simulink model "NonLineare"  (R2020b)
settings: Solver=ode45  StartTime=0.0  StopTime=100  RelTol=1e-6
values from neighbouring files (symbols this model uses):
  alpha = 1    [Assignment7Mat.m]
  C_te = [1 0 0 0]    [Assignment7Mat.m]
  d1_amp = 0.5    [Assignment7Mat.m]
  d1_period = 50    [Assignment7Mat.m]
  F = 1    [Assignment7Mat.m]
  g = 9.81    [Assignment7Mat.m]
  K = -ack*pDesA    [Assignment7Mat.m]
  l = 1    [Assignment7Mat.m]
  L = Gamma - K*Pi    [Assignment7Mat.m]
  M = 1    [Assignment7Mat.m]
  omega = 0.1    [Assignment7Mat.m]
  Q_te = [-1 0 0]    [Assignment7Mat.m]
  x0 = [0 0 0 0]    [Assignment7Mat.m]
settings Model: Creator=Paolo  LastModifiedBy=Paolo

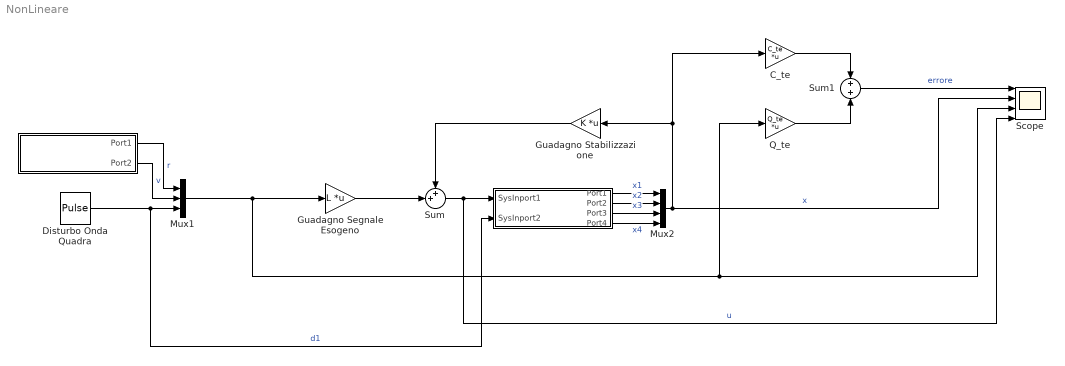
== system NonLineare ==
  "  " : Subsystem  mask(Differential Equation Editor (DEE)){}
      settings: OpenFcn=diffeqed
      mask Display: disp('ModelloNonLineare')
  "   " : Subsystem  mask(Differential Equation Editor (DEE)){}
      settings: OpenFcn=diffeqed
      mask Display: disp('Sistema Esogeno')
  C_te : Gain  Gain=C_te  Multiplication=Matrix(K*u)
  Disturbo Onda Quadra : DiscretePulseGenerator  PulseType=Time based  Amplitude=d1_amp  Period=d1_period  PulseWidth=50
  Guadagno Stabilizzazione : Gain  Gain=K  Multiplication=Matrix(K*u)
  Guadagno Segnale Esogeno : Gain  Gain=L  Multiplication=Matrix(K*u)
  Mux1 : Mux  Inputs=3
  Mux2 : Mux
  Q_te : Gain  Gain=Q_te  Multiplication=Matrix(K*u)
  Scope : Scope  NumInputPorts=4
  Sum : Sum  Inputs=++|
  Sum1 : Sum  Inputs=+|+
  wires:
  Mux2/1 -> C_te/1, Guadagno Stabilizzazione/1, Scope/2  "x"
  "   "/2(Port2) -> Mux1/2  "v"
  Guadagno Stabilizzazione/1 -> Sum/1
  Mux1/1 -> Scope/3, Q_te/1, Guadagno Segnale Esogeno/1
  Guadagno Segnale Esogeno/1 -> Sum/2
  C_te/1 -> Sum1/1
  Sum1/1 -> Scope/1  "errore"
  Sum/1 -> "  "/1(SysInport1), Scope/4  "u"
  Q_te/1 -> Sum1/2
  "   "/1(Port1) -> Mux1/1  "r"
  Disturbo Onda Quadra/1 -> "  "/2(SysInport2), Mux1/3  "d1"
  "  "/1(Port1) -> Mux2/1  "x1"
  "  "/2(Port2) -> Mux2/2  "x2"
  "  "/4(Port4) -> Mux2/4  "x4"
  "  "/3(Port3) -> Mux2/3  "x3"

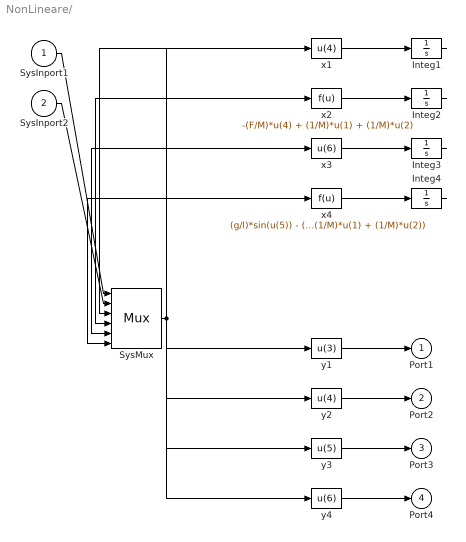
== system NonLineare/   ==
  SysInport1 : Inport
  SysInport2 : Inport  Port=2
  Integ1 : Integrator  InitialCondition=x0(1)
  Integ2 : Integrator  InitialCondition=x0(2)
  Integ3 : Integrator  InitialCondition=x0(3)
  Integ4 : Integrator  InitialCondition=x0(4)
  SysMux : Mux  Inputs=6
  x1 : Fcn  Expr=u(4)
  x2 : Fcn  Expr=-(F/M)*u(4) + (1/M)*u(1) + (1/M)*u(2)
  x3 : Fcn  Expr=u(6)
  x4 : Fcn  Expr=(g/l)*sin(u(5)) - (1/l)*cos(u(5))*(-(F/M)*u(4) + (1/M)*u(1) + (1/M)*u(2))
  y1 : Fcn  Expr=u(3)
  y2 : Fcn  Expr=u(4)
  y3 : Fcn  Expr=u(5)
  y4 : Fcn  Expr=u(6)
  Port1 : Outport
  Port2 : Outport  Port=2
  Port3 : Outport  Port=3
  Port4 : Outport  Port=4
  wires:
  SysInport1/1 -> SysMux/1
  SysInport2/1 -> SysMux/2
  SysMux/1 -> x1/1, x2/1, x3/1, x4/1, y1/1, y2/1, y3/1, y4/1
  x1/1 -> Integ1/1
  Integ1/1 -> SysMux/3
  x2/1 -> Integ2/1
  Integ2/1 -> SysMux/4
  x3/1 -> Integ3/1
  Integ3/1 -> SysMux/5
  x4/1 -> Integ4/1
  Integ4/1 -> SysMux/6
  y1/1 -> Port1/1
  y2/1 -> Port2/1
  y3/1 -> Port3/1
  y4/1 -> Port4/1

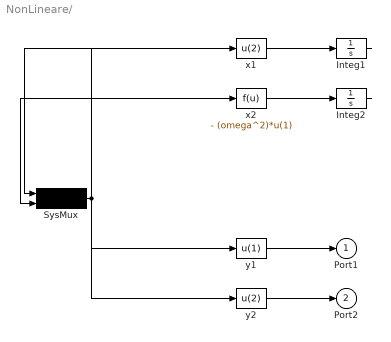
== system NonLineare/    ==
  Integ1 : Integrator
  Integ2 : Integrator  InitialCondition=omega*alpha
  SysMux : Mux  Inputs=2
  x1 : Fcn  Expr=u(2)
  x2 : Fcn  Expr=- (omega^2)*u(1)
  y1 : Fcn  Expr=u(1)
  y2 : Fcn  Expr=u(2)
  Port1 : Outport
  Port2 : Outport  Port=2
  wires:
  SysMux/1 -> x1/1, x2/1, y1/1, y2/1
  x1/1 -> Integ1/1
  Integ1/1 -> SysMux/1
  x2/1 -> Integ2/1
  Integ2/1 -> SysMux/2
  y1/1 -> Port1/1
  y2/1 -> Port2/1
